simulink model "etc_mask4"  (R2022b)
settings: Solver=FixedStepDiscrete  StartTime=0.0  StopTime=10  FixedStep=.01  RelTol=1e-3  EnableMultiTasking=on
PreLoadFcn:
  | % Input step signal
  | t = [0 1 1 10]';
  | u = [0 0 1 1]';
Description:
  | This is my help
settings Model: ParamWorkspaceSource=ReferencedWorkspace  Creator=nicholas  LastModifiedBy=bensweet
settings SolverCC: AlgebraicLoopSolver=TrustRegion
settings DataIOCC: LimitDataPoints=on  LoadExternalInput=on  SaveFormat=Array  ReturnWorkspaceOutputs=off  SignalLoggingName=sigsOut
settings OptimizationCC: DefaultParameterBehavior=Inlined  ExpressionDepthLimit=2147483647  InitFltsAndDblsToZero=on  LifeSpan=inf
settings DebuggingCC: UnconnectedInputMsg=warning  UnconnectedOutputMsg=warning  UnconnectedLineMsg=warning  PregeneratedLibrarySubsystemCodeDiagnostic=none  SFMachineParentedDataDiag=warning
settings HardwareCC: ProdBitPerPointer=32  ProdBitPerSizeT=32  ProdBitPerPtrDiffT=32  ProdLargestAtomicFloat=None  ProdIntDivRoundTo=Undefined  ProdEndianess=Unspecified  ProdWordSize=32  ProdHWDeviceType=32-bit Generic  TargetIntDivRoundTo=Zero  TargetEndianess=BigEndian  TargetHWDeviceType=Motorola PowerPC
settings ModelReferenceCC: EnableRefExpFcnMdlSchedulingChecks=on  PropagateSignalLabelsOutOfModel=off
settings SFSimCC: SimUseLocalCustomCode=off
settings RTWCC: RTWUseLocalCustomCode=off  DLArmComputeVersion=19.05
settings CodeAppCC: StateflowObjectComments=on
settings GRTTargetCC: TargetFcnLib=ansi_tfl_tmw.mat  TargetLangStandard=C89/C90 (ANSI)  CombineOutputUpdateFcns=off  GRTInterface=on
settings ConfigComp: CovMetricSettings=dw  CovSaveCumulativeToWorkspaceVar=on  CovSaveSingleToWorkspaceVar=on  CovExternalEMLEnable=off  CovSFcnEnable=off

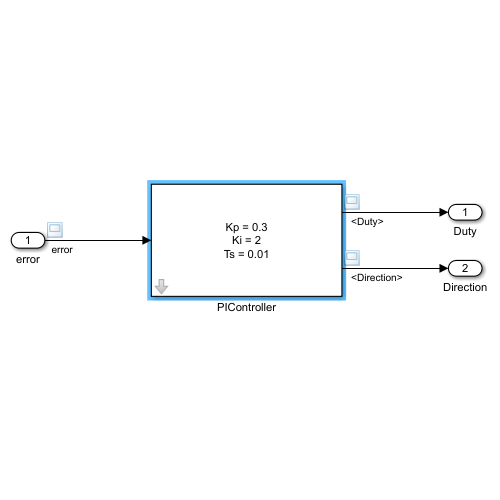
[thumbnail: Simulink's stored preview of the top-level diagram]
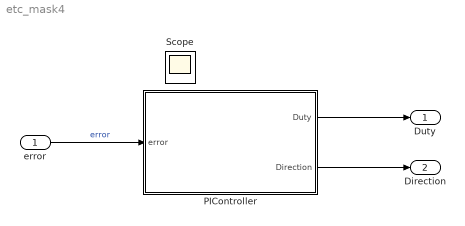
== system etc_mask4 ==
  error : Inport
  PIController : Subsystem  mask(PI Controller){Kp=0.3, Ki=2, Ts=0.01}
      mask prompts: Kp "Proportional Gain (Kp)"; Ki "Integral Gain (Ki)"; Ts "Sample Time (Ts)"
      mask help:
      | This system implements the dynamics of a discrete PI controller with a rate limiter on the integrator.
      | You must specify the proportional gain (Kp), integral gain (Ki), and sample time (Ts) for the system.
      mask init:
      | str1 = "Kp = " + Kp;
      | str2 = "Ki = " + Ki;
      | str3 = "Ts = " + Ts;
      | label = [str1;str2;str3];
      mask Help:
      | This system implements the dynamics of a discrete PI controller with a rate limiter on the integrator.
      | The equations for the system are:  <br /><br />
      | 
      | <b>Y(k) = Yp(k) + Yi(k)</b><br />
      | Yp(k) = Kp*e(k)<br />
      | Yi(k) = Yi(k-1) + Ki*Ts*e(k)<br />
      | -1 < Yi(k) < 1<br /><br />
      | 
      | Define values for Kp, Ki, and Ts for this system.
      mask Display: disp(label)
  Duty : Outport  VectorParamsAs1DForOutWhenUnconnected=off
  Direction : Outport  Port=2  VectorParamsAs1DForOutWhenUnconnected=off
  Scope : Scope
  wires:
  PIController/1(Duty) -> Duty/1
  PIController/2(Direction) -> Direction/1
  error/1 -> PIController/1(error)  "error"

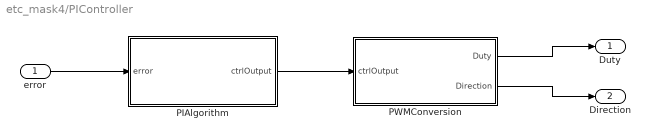
== system etc_mask4/PIController ==
  error : Inport  SampleTime=Ts
  PIAlgorithm : Subsystem
  PWMConversion : Subsystem
  Duty : Outport  VectorParamsAs1DForOutWhenUnconnected=off
  Direction : Outport  Port=2  VectorParamsAs1DForOutWhenUnconnected=off
  wires:
  error/1 -> PIAlgorithm/1(error)
  PWMConversion/1(Duty) -> Duty/1
  PWMConversion/2(Direction) -> Direction/1
  PIAlgorithm/1(ctrlOutput) -> PWMConversion/1(ctrlOutput)

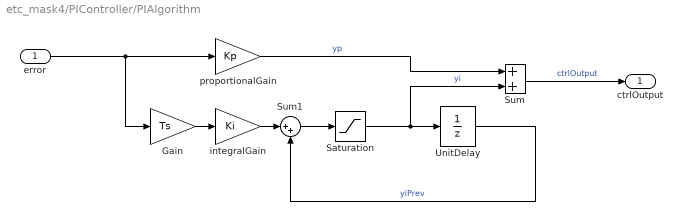
== system etc_mask4/PIController/PIAlgorithm ==
  error : Inport  SampleTime=Ts
      settings: AttributesFormatString=Sample time = %<SampleTime>
  Gain : Gain  Gain=Ts  SaturateOnIntegerOverflow=on  OutDataTypeStr=Inherit: Same as input  ParamDataTypeStr=Inherit: Same as input
  Saturation : Saturate  UpperLimit=1  LowerLimit=-1
      settings: AttributesFormatString=Max: %<UpperLimit>\nMin: %<LowerLimit>
  Sum : Sum  InputSameDT=on  SaturateOnIntegerOverflow=on  OutDataTypeStr=Inherit: Same as first input
  Sum1 : Sum  Inputs=|++  InputSameDT=on  SaturateOnIntegerOverflow=on  OutDataTypeStr=Inherit: Same as first input
  UnitDelay : UnitDelay  SampleTime=Ts  HasFrameUpgradeWarning=on
      settings: AttributesFormatString=yi0 = %<X0>\nSample time = %<SampleTime>
  integralGain : Gain  Gain=Ki  SaturateOnIntegerOverflow=on  OutDataTypeStr=Inherit: Same as input  ParamDataTypeStr=Inherit: Same as input
  proportionalGain : Gain  Gain=Kp  SaturateOnIntegerOverflow=on  OutDataTypeStr=Inherit: Same as input  ParamDataTypeStr=Inherit: Same as input
  ctrlOutput : Outport  VectorParamsAs1DForOutWhenUnconnected=off
  wires:
  proportionalGain/1 -> Sum/1  "yp"
  integralGain/1 -> Sum1/1
  Gain/1 -> integralGain/1
  UnitDelay/1 -> Sum1/2  "yiPrev"
  Sum1/1 -> Saturation/1
  Saturation/1 -> UnitDelay/1, Sum/2  "yi"
  error/1 -> proportionalGain/1, Gain/1
  Sum/1 -> ctrlOutput/1  "ctrlOutput"

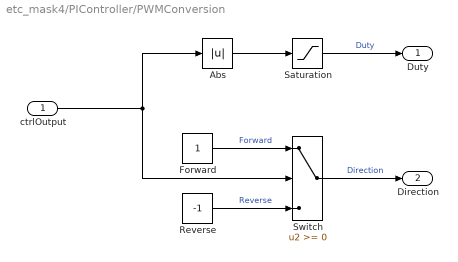
== system etc_mask4/PIController/PWMConversion ==
  ctrlOutput : Inport
  Abs : Abs  SaturateOnIntegerOverflow=off
  Forward : Constant  OutDataTypeStr=double
  Reverse : Constant  Value=-1  OutDataTypeStr=double
  Saturation : Saturate  UpperLimit=1  LowerLimit=0
      settings: AttributesFormatString=%<LowerLimit> < duty < %<UpperLimit>
  Switch : Switch  SaturateOnIntegerOverflow=off  InputSameDT=off
      settings: AttributesFormatString=Criteria: %<Criteria>\nThreshold: %<Threshold>
  Duty : Outport  VectorParamsAs1DForOutWhenUnconnected=off
  Direction : Outport  Port=2  VectorParamsAs1DForOutWhenUnconnected=off
  wires:
  Abs/1 -> Saturation/1
  Saturation/1 -> Duty/1  "Duty"
  Switch/1 -> Direction/1  "Direction"
  Reverse/1 -> Switch/3  "Reverse"
  Forward/1 -> Switch/1  "Forward"
  ctrlOutput/1 -> Switch/2, Abs/1
